simulink model "MBD_WEEK2_QN4"  (R2020b)
settings: Solver=VariableStepAuto  StartTime=0.0  StopTime=1  RelTol=1e-3
values from neighbouring files (symbols this model uses):
  b = 3.5076999999999995E-6    [motor_position_control_variable_data.sldd]
  J = 3.2284E-6    [motor_position_control_variable_data.sldd]
  Kt = 0.0274    [motor_position_control_variable_data.sldd]
  L = 2.75E-6    [motor_position_control_variable_data.sldd]
  R = 4.0    [motor_position_control_variable_data.sldd]
settings Model: DataDictionary=motor_position_control_variable_data.sldd  Creator=dell  LastModifiedBy=dell

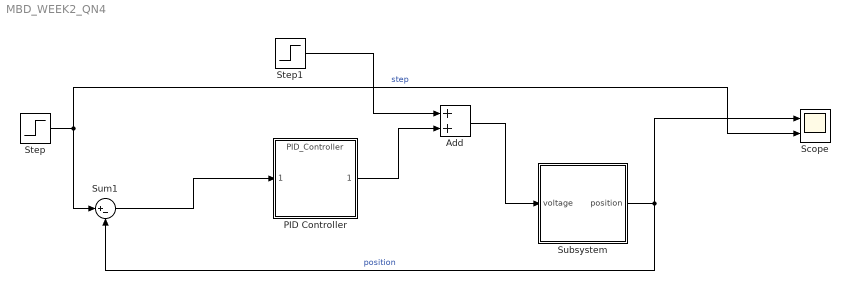
== system MBD_WEEK2_QN4 ==
  Add : Sum
  PID Controller : ModelReference  ModelNameDialog=PID_Controller  SimulationMode=Normal  ModelReferenceVersion=1.12
  Scope : Scope  NumInputPorts=2
  Step : Step  SampleTime=0
  Step1 : Step  Time=0.02  SampleTime=0
  Subsystem : Subsystem
  Sum1 : Sum  Inputs=|+-
  wires:
  Subsystem/1(position) -> Sum1/2, Scope/1  "position"
  Sum1/1 -> PID Controller/1
  Step/1 -> Sum1/1, Scope/2  "step"
  PID Controller/1 -> Add/2
  Add/1 -> Subsystem/1(voltage)
  Step1/1 -> Add/1

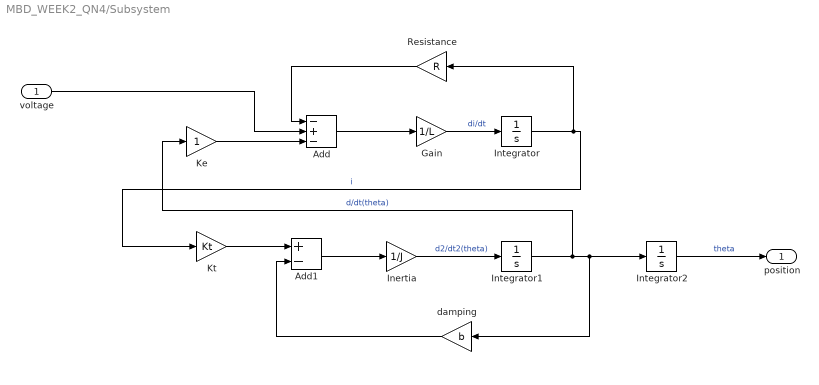
== system MBD_WEEK2_QN4/Subsystem ==
  voltage : Inport
  Add : Sum  Inputs=-+-
  Add1 : Sum  Inputs=+-
  Gain : Gain  Gain=1/L
  Inertia : Gain  Gain=1/J
  Integrator : Integrator
  Integrator1 : Integrator
  Integrator2 : Integrator
  Ke : Gain
  Kt : Gain  Gain=Kt
  Resistance : Gain  Gain=R
  damping : Gain  Gain=b
  position : Outport
  wires:
  Resistance/1 -> Add/1
  Integrator/1 -> Resistance/1, Kt/1  "i"
  Integrator2/1 -> position/1  "theta"
  Inertia/1 -> Integrator1/1  "d2/dt2(theta)"
  Add/1 -> Gain/1
  Ke/1 -> Add/3
  Integrator1/1 -> Ke/1, damping/1, Integrator2/1  "d/dt(theta)"
  Gain/1 -> Integrator/1  "di/dt"
  Add1/1 -> Inertia/1
  damping/1 -> Add1/2
  Kt/1 -> Add1/1
  voltage/1 -> Add/2
